simulink library "Gravity_Lib"  (Simulink 8.0)
settings: Solver=ode45  SolverMode=SingleTasking  StartTime=0.0  StopTime=10.0  RelTol=1e-3
values from neighbouring files (symbols this model uses):
  AC = miniMUTT_config    [UAV_config.m]    (also in UAV_modelconfig.mat = )
libraries: simulink x1
settings Model: Creator=Paul Freeman  LastModifiedBy=brtaylor

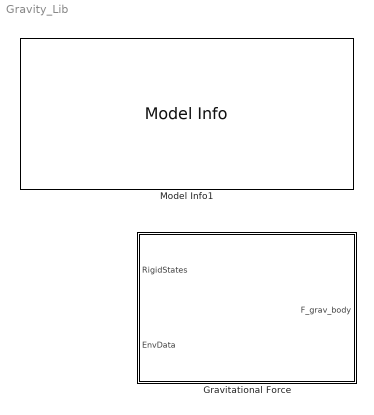
== system Gravity_Lib ==
  "Gravitational Force " : Subsystem
  Model Info1 : simulink/Model-Wide Utilities/Model Info  InitialBlockCM=None  BlockCM=None  Frame=on  DisplayStringWithTags=|  HorizontalTextAlignment=Left  LeftAlignmentValue=0.02  SourceBlockDiagram=Gravity_Lib  TagMaxNumber=20
      | MODEL INFORMATION
      | Gravitational Force Library
      | 
      | University of Minnesota
      | Aerospace Engineering and Mechanics
      | Copyright 2011 Regents of the University of Minnesota. All rights reserved.
      | 
      | == SVN Info ==
      | %<ModelVersion>
      | Last modified by %<LastModifiedBy> on %<LastModificationDate>

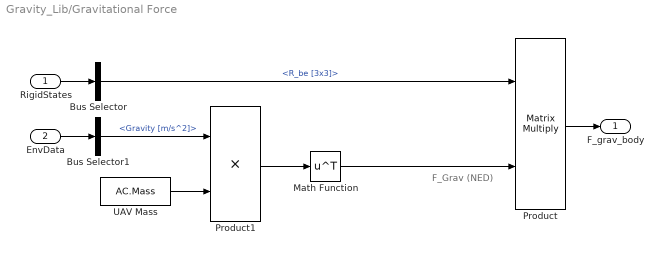
== system Gravity_Lib/Gravitational Force  ==
  note: F_Grav (NED)
  RigidStates : Inport
  EnvData : Inport  Port=2
  Bus Selector : BusSelector  OutputSignals=R_be [3x3]
  Bus Selector1 : BusSelector  OutputSignals=Gravity [m/s^2]
  Math Function : Math  Operator=transpose  SaturateOnIntegerOverflow=on
  Product : Product  Multiplication=Matrix(*)  SaturateOnIntegerOverflow=on  RndMeth=Zero  InputSameDT=on  OutDataTypeStr=Inherit: Same as first input
  Product1 : Product  SaturateOnIntegerOverflow=on  RndMeth=Zero  InputSameDT=on  OutDataTypeStr=Inherit: Same as first input
  UAV Mass : Constant  Value=AC.Mass
  F_grav_body : Outport
  wires:
  Product/1 -> F_grav_body/1
  Bus Selector/1 -> Product/1  "<R_be [3x3]>"
  RigidStates/1 -> Bus Selector/1
  EnvData/1 -> Bus Selector1/1
  Bus Selector1/1 -> Product1/1  "<Gravity [m/s^2]>"
  UAV Mass/1 -> Product1/2
  Product1/1 -> Math Function/1
  Math Function/1 -> Product/2
